simulink model "Slew_Constant_target"  (R2026a)
settings: Solver=VariableStepAuto  StopTime=40000
values from neighbouring files (symbols this model uses):
  c = 2 * zeta * omega_n    (= 0.1)    [inizializzazione.m]
  J = [3190 0 0; 0 3790 0; 0 0 5672]    [inizializzazione.m]
  kappa = omega_n^2    (= 0.0025)    [inizializzazione.m]
  q_target = [q1; q2; q3; q4]    [inizializzazione.m]
  state_0 = [q_true_0; w_true_0]    [inizializzazione.m]
  tau_m = 0.106    [inizializzazione.m]
  theta_deg = 45    [inizializzazione.m]
settings Model: Creator=mario  LastModifiedBy=mario

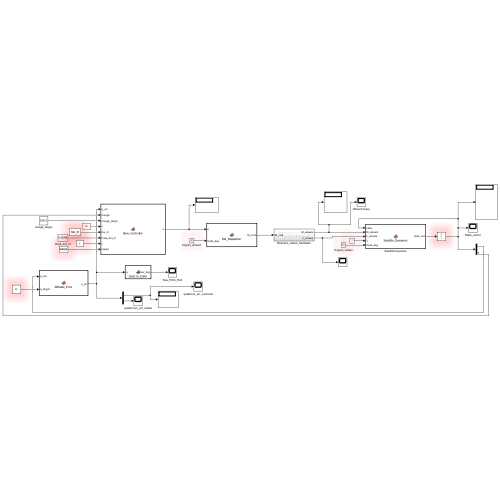
[thumbnail: Simulink's stored preview of the top-level diagram]
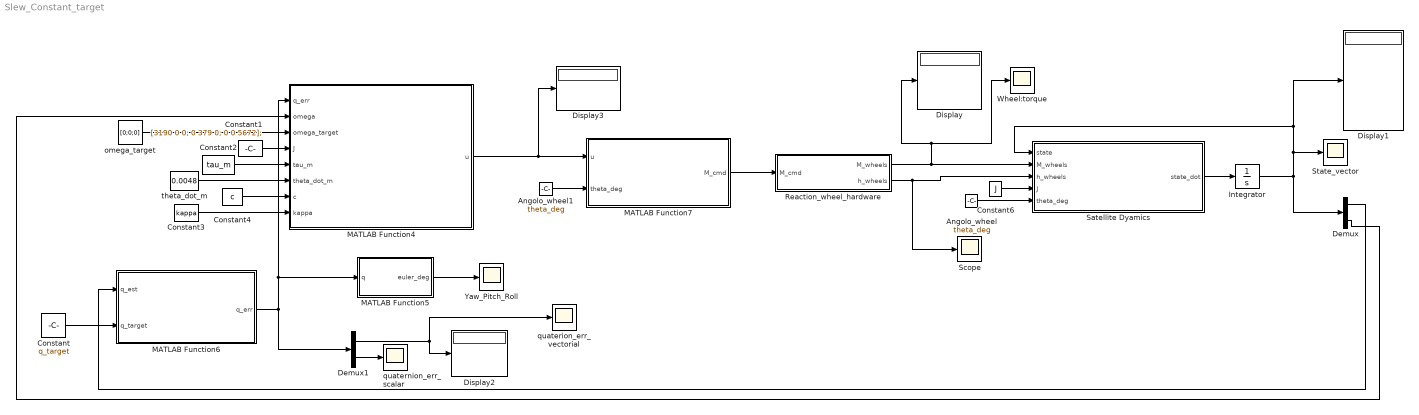
== system Slew_Constant_target ==
  Angolo_wheel : Constant  Value=theta_deg
  Angolo_wheel1 : Constant  Value=theta_deg
  Constant : Constant  Value=q_target
  Constant1 : Constant  Value=[3190 0 0; 0 379 0; 0 0 5672];
  Constant2 : Constant  Value=tau_m
  Constant3 : Constant  Value=kappa
  Constant4 : Constant  Value=c
  Constant6 : Constant  Value=J
  Demux : Demux  Outputs=2
  Demux1 : Demux  Outputs=[3 1]
  Display{,1..3} (4 alike) : Display
  Integrator : Integrator  InitialCondition=state_0
  MATLAB Function4 : MATLAB Function  TreatAsAtomicUnit=on
  MATLAB Function5 : MATLAB Function  TreatAsAtomicUnit=on
  MATLAB Function6 : MATLAB Function  TreatAsAtomicUnit=on
  MATLAB Function7 : MATLAB Function  TreatAsAtomicUnit=on
  Reaction_wheel_hardware : Subsystem
  Satellite Dyamics : MATLAB Function  TreatAsAtomicUnit=on
  Scope : Scope
      settings: DataLoggingVariableName=ScopeData5
  State_vector : Scope
      settings: ActiveDisplayYMinimum=-0.20980740065652753  ActiveDisplayYMaximum=0.16165384213934825
  Wheel:torque : Scope
      settings: ActiveDisplayYMinimum=-0.19667273357596288  ActiveDisplayYMaximum=0.322070588683968
  Yaw_Pitch_Roll : Scope
      settings: ActiveDisplayYMinimum=-19.760680553123535  ActiveDisplayYMaximum=11.07233486493166  DataLoggingVariableName=ScopeData2
  omega_target : Constant  Value=[0;0;0]
  quaterion_err_vectorial : Scope
      settings: ActiveDisplayYMinimum=-0.14741933252380829  ActiveDisplayYMaximum=-0.12086964198147464  DataLoggingVariableName=ScopeData3
  quaternion_err_scalar : Scope
      settings: ActiveDisplayYMinimum=-0.87381284022924977  ActiveDisplayYMaximum=1.9707894578453811  DataLoggingVariableName=ScopeData4
  theta_dot_m : Constant  Value=0.0048
  wires:
  Reaction_wheel_hardware/2(h_wheels) -> Scope/1, Satellite Dyamics/3(h_wheels)
  Satellite Dyamics/1(state_dot) -> Integrator/1
  theta_dot_m/1 -> MATLAB Function4/6(theta_dot_m)
  Demux/2 -> MATLAB Function4/2(omega)
  Demux/1 -> MATLAB Function6/1(q_est)
  Constant4/1 -> MATLAB Function4/7(c)
  Constant3/1 -> MATLAB Function4/8(kappa)
  Constant2/1 -> MATLAB Function4/5(tau_m)
  MATLAB Function5/1(euler_deg) -> Yaw_Pitch_Roll/1
  Demux1/2 -> quaternion_err_scalar/1
  MATLAB Function4/1(u) -> MATLAB Function7/1(u), Display3/1
  Constant1/1 -> MATLAB Function4/4(J)
  Constant6/1 -> Satellite Dyamics/4(J)
  MATLAB Function7/1(M_cmd) -> Reaction_wheel_hardware/1(M_cmd)
  Reaction_wheel_hardware/1(M_wheels) -> Display/1, Wheel:torque/1, Satellite Dyamics/2(M_wheels)
  Angolo_wheel/1 -> Satellite Dyamics/5(theta_deg)
  Angolo_wheel1/1 -> MATLAB Function7/2(theta_deg)
  MATLAB Function6/1(q_err) -> MATLAB Function4/1(q_err), MATLAB Function5/1(q), Demux1/1
  Demux1/1 -> Display2/1, quaterion_err_vectorial/1
  Integrator/1 -> Demux/1, State_vector/1, Display1/1, Satellite Dyamics/1(state)
  Constant/1 -> MATLAB Function6/2(q_target)
  omega_target/1 -> MATLAB Function4/3(omega_target)

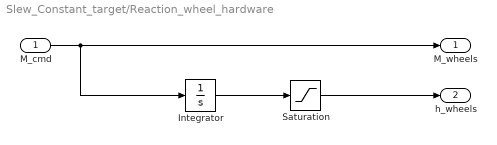
== system Slew_Constant_target/Reaction_wheel_hardware ==
  M_cmd : Inport  PortDimensions=4
  Integrator : Integrator  InitialCondition=[0; 0; 0; 0]  LimitOutput=on  UpperSaturationLimit=12  LowerSaturationLimit=-12
  Saturation : Saturate  UpperLimit=50  LowerLimit=-50
  M_wheels : Outport
  h_wheels : Outport  Port=2
  wires:
  M_cmd/1 -> Integrator/1, M_wheels/1
  Integrator/1 -> Saturation/1
  Saturation/1 -> h_wheels/1

== matlab function Slew_Constant_target/Satellite Dyamics ==
  data: state input; state_dot output; M_wheels input; h_wheels input; J input; theta_deg input
function state_dot = Satellite_Dynamics(state, M_wheels, h_wheels, J, theta_deg)

    %% 0. MESSA IN SICUREZZA DELLE DIMENSIONI (Evita gli errori di compilazione Simulink)
    % Dichiariamo subito la dimensione dell'uscita
    state_dot = zeros(7,1); 
    
    % Forziamo tutti i segnali in ingresso a essere vettori colonna (Nx1)
    state = state(:);
    M_wheels = M_wheels(:);
    h_wheels = h_wheels(:);
    
    % Assicuriamoci che l'angolo sia uno scalare
    theta_deg = theta_deg(1);

    %% 1. ESTRAZIONE DELLO STATO
    % Quaternione (Convenzione Scalar-Last)
    q = state(1:4); 
    % Velocità angolare [rad/s]
    w = state(5:7); 

    %% 2. MATRICE DELLA GEOMETRIA DELLE RUOTE
    theta = theta_deg * (pi/180); 
    
    % Matrice di attuazione Aw per la configurazione a 4 ruote inclinate
    Aw = [ cos(theta),      0,       -cos(theta),      0;
           sin(theta),  sin(theta),   sin(theta),  sin(theta);
               0,      -cos(theta),       0,       cos(theta)];
               
    % Proiezione dai 4 assi delle ruote ai 3 assi del corpo
    M_contr = Aw * M_wheels; 
    h_w_contr = Aw * h_wheels; 

    %% 3. DINAMICA ROTAZIONALE (Equazioni di Eulero Accoppiate)
    skew_w = [   0,   -w(3),   w(2);
               w(3),     0,  -w(1);
              -w(2),   w(1),     0 ];
              % bigogna inserire il contributo di gravity gradient e
              % external torque nella formula sotto
              
    w_dot = J \ (-M_contr - skew_w * (J * w + h_w_contr)); 

    %% 4. CINEMATICA D'ASSETTO (Derivata del Quaternione)
    q_v = q(1:3); 
    q_s = q(4);   
    
    q_v_dot = -0.5 * skew_w * q_v + 0.5 * q_s * w;
    q_s_dot = -0.5 * w' * q_v;
    
    q_dot = [q_v_dot; q_s_dot];

    %% 5. ASSEMBLAGGIO DELL'USCITA
    state_dot = [q_dot; w_dot];
    % Calcolo dell'errore di norma del quaternione
    norm_err = 1 - (q(1)^2 + q(2)^2 + q(3)^2 + q(4)^2);
    k_norm = 0.05; % Abbassato da 10 per garantire stabilità numerica

    % Aggiungiamo il termine di Baumgarte alla derivata
    q_dot = [q_v_dot; q_s_dot] + k_norm * norm_err * q;

    % Vettore di stato derivato in uscita
    state_dot = [q_dot; w_dot];
end

== matlab function Slew_Constant_target/MATLAB Function4 ==
  data: q_err input; u output; omega input; omega_target input; J input; tau_m input; theta_dot_m input; c input; kappa input
function u = Slew_Controller(q_err, omega, omega_target, J, tau_m, theta_dot_m, c, kappa)
    % 1. ERRORE DI ASSETTO E DI VELOCITÀ RELATIVA
    q_e = q_err(1:3);
    norm_qe = norm(q_e);
    
    % La velocità relativa al bersaglio orbitale (Inseguimento)
    delta_omega = omega - omega_target;

    % Sicurezza: se l'errore è microscopico, spegni i motori e risparmia energia
    if norm_qe < 1e-6
        u = [0; 0; 0];
        return;
    end

    % 2. CALCOLO DEI GUADAGNI DEL CONTROLLORE DI KJELLBERG
    % C è il "freno" (Azione derivativa)
    C = c * J;

    % K è la "molla" proporzionale per ogni asse
    k1 = c * (abs(q_e(1)) / norm_qe) * theta_dot_m;
    k2 = c * (abs(q_e(2)) / norm_qe) * theta_dot_m;
    k3 = c * (abs(q_e(3)) / norm_qe) * theta_dot_m;
    K = diag([k1, k2, k3]) * J;

    % 3. CALCOLO DELLA VELOCITÀ DESIDERATA (Senza divisioni per zero)
    % Uso 'epsilon' per evitare che il calcolo esploda e per addolcire la frenata
    epsilon = 1e-3; 
    coeff = (kappa * norm_qe) / (c * theta_dot_m);
    
    v_in = zeros(3,1);
    v_in(1) = coeff * (q_e(1) / (abs(q_e(1)) + epsilon));
    v_in(2) = coeff * (q_e(2) / (abs(q_e(2)) + epsilon));
    v_in(3) = coeff * (q_e(3) / (abs(q_e(3)) + epsilon));

    % 4. SATURAZIONE INTERNA
    % Taglia la richiesta matematica se l'errore iniziale di 140° è troppo grande
    %v_sat = max(min(v_in, 1), -1);
    v_sat = tanh(v_in);

    % 5. COPPIA TEORICA BODY (Molla proporzionale + Freno derivativo)
    tau = K * v_sat + C * delta_omega;
    
    % --- NUOVO PUNTO 6: SATURAZIONE SULLE RUOTE ---
    % Calcola in anticipo la coppia che verrebbe richiesta alle 4 ruote

    % tau_wheels_raw = W_pinv * tau; 
    % 
    % % Calcola il fattore di saturazione sigma usando i valori delle ruote reali!
    % sigma = max(abs(tau_wheels_raw) / tau_m);

    % Calcola il fattore di saturazione sigma usando i valori delle ruote reali!
    sigma = max(abs(tau) / tau_m);
    
    % Se almeno una ruota supera tau_m, sigma sarà > 1.
    % Riduciamo la coppia BODY proporzionalmente per mantenere la traiettoria (Eigenaxis)
    if sigma > 1
        u = tau / sigma;   % Applica la riduzione vettoriale
    else
        u = tau;
    end
end

== matlab function Slew_Constant_target/MATLAB Function5 ==
  data: q input; euler_deg output
function euler_deg = Quat_to_Euler(q)
% INGRESSO: q (Quaternione 4x1, convenzione Scalar-Last)
% USCITA: euler_deg (Vettore 3x1 con [Roll; Pitch; Yaw] in GRADI)

% 1. Estrazione degli elementi del quaternione
q1 = q(1);
q2 = q(2);
q3 = q(3);
q4 = q(4); % Elemento scalare

% 2. Calcolo dei soli elementi della Matrice di Rotazione (DCM) necessari
% Formule basate sulla trasformazione Quaternione -> DCM
M11 = q1^2 - q2^2 - q3^2 + q4^2;
M12 = 2 * (q1*q2 + q3*q4);
M13 = 2 * (q1*q3 - q2*q4);
M23 = 2 * (q2*q3 + q1*q4);
M33 = -q1^2 - q2^2 + q3^2 + q4^2;

% 3. Estrazione degli angoli di Eulero (Sequenza 3-2-1)

% ROLLIO (Roll / Phi) - Rotazione attorno asse X
roll = atan2(M23, M33);

% BECCHEGGIO (Pitch / Theta) - Rotazione attorno asse Y
% Aggiungiamo una protezione numerica per evitare che errori di
% arrotondamento portino l'argomento di asin fuori da [-1, 1],
% il che genererebbe numeri complessi e manderebbe in blocco Simulink.
sin_p = -M13;
sin_p = max(min(sin_p, 1), -1);
pitch = asin(sin_p);

% IMBARDATA (Yaw / Psi) - Rotazione attorno asse Z
yaw = atan2(M12, M11);

% 4. Conversione in GRADI e assemblaggio del vettore in uscita
euler_deg = [roll; pitch; yaw] * (180 / pi);
end

== matlab function Slew_Constant_target/MATLAB Function6 ==
  data: q_est input size=[4 1]; q_err output size=[4 1]; q_target input size=[4 1]
function q_err = Attitude_Error(q_est, q_target)
    % 1. Calcola l'inverso del quaternione target (Convenzione Scalar-Last)
    % L'inverso di un quaternione unitario coincide con il suo coniugato
    q_target_inv = [-q_target(1:3); q_target(4)];
    
    % 2. Moltiplicazione quaternionica: q_target_inv (X) q_est
    % Applichiamo rigorosamente la formula del prodotto per la convenzione Scalar-Last
    q_err_vec = q_est(4)*q_target_inv(1:3) + q_target_inv(4)*q_est(1:3) - cross(q_est(1:3), q_target_inv(1:3));
    q_err_sca = q_target_inv(4)*q_est(4) - dot(q_target_inv(1:3), q_est(1:3));
    
    q_err = [q_err_vec; q_err_sca];
    
    % 3. Forziamo la rotazione minima (Shortest path)
    % Evita che il satellite compia una rotazione maggiore di 180 gradi
    if q_err(4) < 0
        q_err = -q_err;
    end
end

== matlab function Slew_Constant_target/MATLAB Function7 ==
  data: u input; M_cmd output; theta_deg input
function M_cmd = RW_Dispatcher(u, theta_deg)
    % u: Coppia desiderata sui 3 assi del satellite (dal Slew_Controller)
    % theta: angolo di inclinazione delle ruote (es. 45 * pi/180)
    theta = theta_deg * (pi/180); 
    % Matrice di configurazione hardware a 4 ruote inclinate
    Aw = [cos(theta),          0, -cos(theta),           0;
          sin(theta), sin(theta),  sin(theta),  sin(theta);
                   0, -cos(theta),          0,  cos(theta)];
          
    % Calcolo della Right Pseudoinverse
    Aw_pinv = pinv(Aw);
    
    % Distribuzione della coppia: minimizza l'energia spesa dalle 4 ruote
    M_cmd = Aw_pinv * (-u);
end
